simulink model "decimator_model"  (R2021a)
settings: Solver=FixedStepDiscrete  StartTime=0.0  StopTime=1000  FixedStep=1  RelTol=1e-3
libraries: simulink x2
settings Model: Creator=user  LastModifiedBy=user

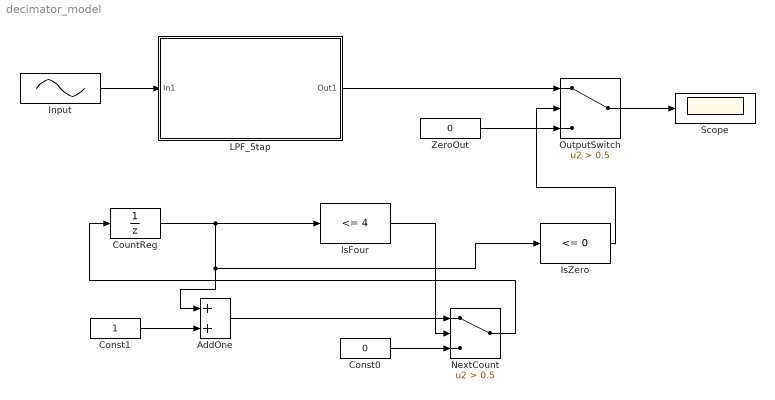
== system decimator_model ==
  AddOne : Sum
  Const0 : Constant  Value=0
  Const1 : Constant
  CountReg : UnitDelay  HasFrameUpgradeWarning=on
  Input : Sin  Frequency=0.01  SampleTime=1
  IsFour : simulink/Logic and Bit Operations/Compare To Constant  relop=<=  const=4  OutDataTypeStr=boolean
  IsZero : simulink/Logic and Bit Operations/Compare To Constant  relop=<=  const=0  OutDataTypeStr=boolean
  LPF_5tap : Subsystem
  NextCount : Switch  Criteria=u2 > Threshold  Threshold=0.5
  OutputSwitch : Switch  Criteria=u2 > Threshold  Threshold=0.5
  Scope : Scope
  ZeroOut : Constant  Value=0
  wires:
  CountReg/1 -> AddOne/1, IsZero/1, IsFour/1
  Const1/1 -> AddOne/2
  AddOne/1 -> NextCount/1
  IsFour/1 -> NextCount/2
  Const0/1 -> NextCount/3
  NextCount/1 -> CountReg/1
  Input/1 -> LPF_5tap/1(In1)
  LPF_5tap/1(Out1) -> OutputSwitch/1
  IsZero/1 -> OutputSwitch/2
  ZeroOut/1 -> OutputSwitch/3
  OutputSwitch/1 -> Scope/1

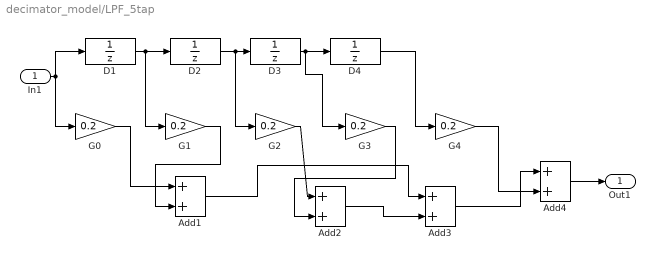
== system decimator_model/LPF_5tap ==
  In1 : Inport
  Add{1..4} (4 alike) : Sum
  D{1..4} (4 alike) : UnitDelay  HasFrameUpgradeWarning=on
  G{0..4} (5 alike) : Gain  Gain=0.2
  Out1 : Outport
  wires:
  In1/1 -> D1/1, G0/1
  D1/1 -> G1/1, D2/1
  D2/1 -> G2/1, D3/1
  D3/1 -> G3/1, D4/1
  D4/1 -> G4/1
  G0/1 -> Add1/1
  G1/1 -> Add1/2
  G2/1 -> Add2/1
  G3/1 -> Add2/2
  Add1/1 -> Add3/1
  Add2/1 -> Add3/2
  Add3/1 -> Add4/1
  G4/1 -> Add4/2
  Add4/1 -> Out1/1
